simulink model "New_Controller"  (R2020b)
settings: Solver=VariableStepAuto  StartTime=0.0  StopTime=100  MaxStep=0.1  RelTol=1e-3
libraries: pid_lib x1
settings Model: Creator=Inver  LastModifiedBy=Inver

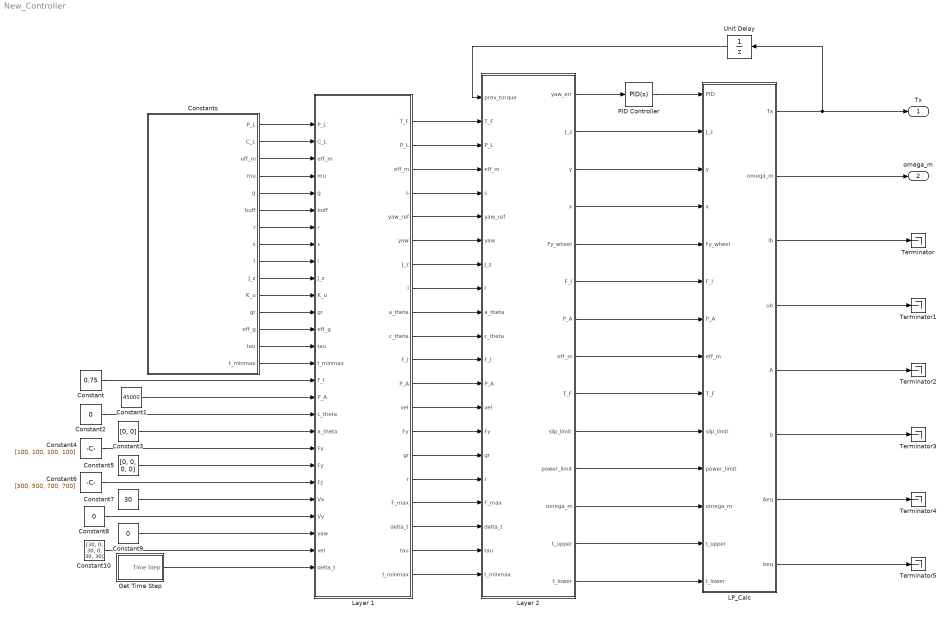
== system New_Controller ==
  Constant : Constant  Value=0.75
  Constant1 : Constant  Value=45000
  Constant10 : Constant  Value=[30, 0, 30, 0, 30, 30]
  Constant2 : Constant  Value=0
  Constant3 : Constant  Value=[0, 0]
  Constant4 : Constant  Value=[100, 100, 100, 100]
  Constant5 : Constant  Value=[0, 0, 0, 0]  VectorParams1D=off
  Constant6 : Constant  Value=[500, 500, 700, 700]
  Constant7 : Constant  Value=30
  Constant8 : Constant  Value=0
  Constant9 : Constant  Value=0
  "Constants " : MATLAB Function  TreatAsAtomicUnit=on
  Get Time Step : Subsystem
  "LP_Calc " : MATLAB Function  TreatAsAtomicUnit=on
  Layer 1 : MATLAB Function  TreatAsAtomicUnit=on
  Layer 2 : MATLAB Function  TreatAsAtomicUnit=on
  PID Controller : pid_lib/PID Controller  Controller=PID  Form=Parallel  TimeDomain=Continuous-time  UseExternalTs=off  SampleTime=-1  IntegratorMethod=Forward Euler  FilterMethod=Forward Euler  ControllerParametersSource=internal  P=40  I=3  D=0  UseFilter=on  N=100  TunerSelectOption=Transfer Function Based (PID Tuner App)  InitialConditionSource=internal  InitialConditionForIntegrator=0  InitialConditionForFilter=0  DifferentiatorICPrevScaledInput=0  ExternalReset=none  TrackingMode=off  Kt=1  LimitOutput=on  SatLimitsSource=internal  UpperSaturationLimit=inf  LowerSaturationLimit=-inf  LinearizeAsGain=on  AntiWindupMode=back-calculation  Kb=1  POutMin=[]  POutMax=[]  IOutMin=[]  IOutMax=[]  DOutMin=[]  DOutMax=[]  NOutMin=[]  NOutMax=[]  SumOutMin=[]  SumOutMax=[]  SaturationOutMin=[]  SaturationOutMax=[]  PParamMin=[]  PParamMax=[]  IParamMin=[]  IParamMax=[]  DParamMin=[]  DParamMax=[]  NParamMin=[]  NParamMax=[]  KbParamMin=[]  KbParamMax=[]  KtParamMin=[]  KtParamMax=[]  KbOutMin=[]  KbOutMax=[]  KtOutMin=[]  KtOutMax=[]  IntegratorOutMin=[]  IntegratorOutMax=[]  FilterOutMin=[]  FilterOutMax=[]  SumI1OutMin=[]  SumI1OutMax=[]  SumI2OutMin=[]  SumI2OutMax=[]  SumI3OutMin=[]  SumI3OutMax=[]  SumI4OutMin=[]  SumI4OutMax=[]  SumDOutMin=[]  SumDOutMax=[]  DifferentiatorOutMin=[]  DifferentiatorOutMax=[]  FilterDiffOutCoefMin=[]  FilterDiffOutCoefMax=[]  ReciprocalOutMin=[]  ReciprocalOutMax=[]  SumDenOutMin=[]  SumDenOutMax=[]  SumNumOutMin=[]  SumNumOutMax=[]  DivideOutMin=[]  DivideOutMax=[]  UdiffTsProdOutMin=[]  UdiffTsProdOutMax=[]  NTsProdOutMin=[]  NTsProdOutMax=[]  UintegralTsProdOutMin=[]  UintegralTsProdOutMax=[]  UngainTsProdOutMin=[]  UngainTsProdOutMax=[]  IntegratorContinuousStateAttributes=''  IntegratorStateMustResolveToSignalObject=off  IntegratorRTWStateStorageClass=Auto  FilterContinuousStateAttributes=''  FilterStateMustResolveToSignalObject=off  FilterRTWStateStorageClass=Auto  ParallelPVariant=InternalParameters  IdealPVariant=Disabled  IVariant=InternalParameters  DVariant=InternalParameters  IntegratorVariant=Continuous  SatVariant=Enabled  AWVariant=BackCalculation  PCopyVariant=Disabled  TRVariant=Disabled  FdbkBlocksVariant=Forward  IdealPFdbkVariant=Disabled  SatFdbkVariant=Disabled  DerivativeFilterVariant=ContFilter  NVariant=InternalParameters  NCopyVariant=Disabled  FilterICVariant=InternalICsFilter  IntegratorICVariant=InternalICs  ExternalResetVariant=Disabled  TRSumVariant=Passthrough  SumFdbkVariant=Disabled  SumVariant=Sum_PID  TsampFilterVariant=InternalTs  TsampNgainVariant=Passthrough  TsampIntegralVariant=Passthrough  ExternalSaturationOutDataTypeStr=Inherit: Same as second input
  Terminator{,1..5} (6 alike) : Terminator
  Unit Delay : UnitDelay  InitialCondition=[0; 0; 0; 0]  SampleTime=-1  HasFrameUpgradeWarning=on
  Tx : Outport
  omega_m : Outport  Port=2
  wires:
  Layer 1/15(gr) -> Layer 2/16(gr)
  Layer 1/14(Fy) -> Layer 2/15(Fy)
  "LP_Calc "/1(Tx) -> Unit Delay/1, Tx/1
  Layer 2/12(omega_m) -> "LP_Calc "/12("omega_m ")
  "Constants "/6(buff) -> Layer 1/6(buff)
  "Constants "/4(mu) -> Layer 1/4(mu)
  Layer 2/8(eff_m) -> "LP_Calc "/8(eff_m)
  Layer 2/13(t_upper) -> "LP_Calc "/13(t_upper)
  "LP_Calc "/7(Aeq) -> Terminator4/1
  "LP_Calc "/3(lb) -> Terminator/1
  "Constants "/3(eff_m) -> Layer 1/3("eff_m ")
  Layer 2/7(P_A) -> "LP_Calc "/7(P_A)
  "LP_Calc "/5(A) -> Terminator2/1
  Constant7/1 -> Layer 1/23(Vx)
  "LP_Calc "/6(b) -> Terminator3/1
  Layer 2/6(F_I) -> "LP_Calc "/6(F_I)
  Layer 2/10(slip_limit) -> "LP_Calc "/10(slip_limit)
  Layer 1/9(a_theta) -> Layer 2/10(a_theta)
  Layer 2/3(y) -> "LP_Calc "/3(y)
  "Constants "/13(eff_g) -> Layer 1/13(eff_g)
  "Constants "/11(K_u) -> Layer 1/11(K_u)
  Get Time Step/1(Time Step) -> Layer 1/27("delta_t ")
  "Constants "/14(tau) -> Layer 1/14("tau ")
  Constant2/1 -> Layer 1/18("c_theta ")
  Constant/1 -> Layer 1/16("F_I ")
  "LP_Calc "/2(omega_m) -> omega_m/1
  "Constants "/8(s) -> Layer 1/8("s ")
  Layer 1/3(eff_m) -> Layer 2/4("eff_m ")
  Layer 1/13(vel) -> Layer 2/14(vel)
  Constant4/1 -> Layer 1/20(Fx)
  Layer 1/20(t_minmax) -> Layer 2/21(t_minmax)
  Constant10/1 -> Layer 1/26("vel ")
  Layer 1/6(yaw) -> Layer 2/7(yaw)
  Layer 2/5(Fy_wheel) -> "LP_Calc "/5(Fy_wheel)
  Layer 1/4(s) -> Layer 2/5(s)
  Layer 2/9(T_F) -> "LP_Calc "/9(T_F)
  Layer 1/11(F_I) -> Layer 2/12("F_I ")
  "Constants "/12(gr) -> Layer 1/12("gr ")
  Constant3/1 -> Layer 1/19("a_theta ")
  "LP_Calc "/8(beq) -> Terminator5/1
  Layer 1/12(P_A) -> Layer 2/13("P_A ")
  "Constants "/1(P_L) -> Layer 1/1("P_L ")
  Unit Delay/1 -> Layer 2/1(prev_torque)
  Layer 1/7(J_z) -> Layer 2/8("J_z ")
  "Constants "/10(J_z) -> Layer 1/10("J_z ")
  Layer 2/2(J_z) -> "LP_Calc "/2(J_z)
  "Constants "/9(l) -> Layer 1/9("l ")
  Constant9/1 -> Layer 1/25("yaw ")
  Layer 1/5(yaw_ref) -> Layer 2/6(yaw_ref)
  "LP_Calc "/4(ub) -> Terminator1/1
  Constant1/1 -> Layer 1/17("P_A ")
  Layer 1/17(F_max) -> Layer 2/18(F_max)
  "Constants "/7(r) -> Layer 1/7("r ")
  Layer 1/16(r) -> Layer 2/17(r)
  Layer 2/14(t_lower) -> "LP_Calc "/14(t_lower)
  Layer 1/10(c_theta) -> Layer 2/11(c_theta)
  Constant5/1 -> Layer 1/21("Fy ")
  Layer 1/2(P_L) -> Layer 2/3(P_L)
  Constant6/1 -> Layer 1/22(Fz)
  "Constants "/5(g) -> Layer 1/5(g)
  Constant8/1 -> Layer 1/24(Vy)
  Layer 2/1(yaw_err) -> PID Controller/1
  "Constants "/2(C_L) -> Layer 1/2(C_L)
  Layer 1/18(delta_t) -> Layer 2/19(delta_t)
  "Constants "/15(t_minmax) -> Layer 1/15("t_minmax ")
  Layer 1/8(l) -> Layer 2/9(l)
  Layer 2/4(x) -> "LP_Calc "/4(x)
  Layer 1/19(tau) -> Layer 2/20(tau)
  Layer 2/11(power_limit) -> "LP_Calc "/11(power_limit)
  Layer 1/1(T_F) -> Layer 2/2("T_F ")
  PID Controller/1 -> "LP_Calc "/1(PID)

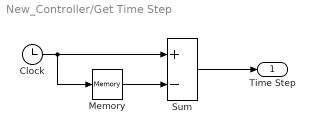
== system New_Controller/Get Time Step ==
  Clock : Clock
  Memory : Memory
  Sum : Sum  Inputs=+-
  Time Step : Outport
  wires:
  Memory/1 -> Sum/2
  Clock/1 -> Sum/1, Memory/1
  Sum/1 -> Time Step/1

== matlab function New_Controller/Layer 2 ==
  data: prev_torque input; yaw_err output; J_z output; T_F input; P_L input; eff_m input; s input; yaw_ref input; yaw input; J_z input; l input; a_theta input; c_theta input; F_I input; P_A input; vel input; Fy input; gr input; r input; F_max input; y output; x output; Fy_wheel output; F_I output; P_A output; eff_m output; T_F output; slip_limit output; power_limit output; omega_m output size=[1 4]; t_upper output; delta_t input; tau input; t_minmax input; t_lower output
function [yaw_err, J_z, y, x, Fy_wheel, F_I, P_A, eff_m, T_F, slip_limit, power_limit, omega_m, t_upper, t_lower] = Layer_2(prev_torque, T_F, P_L, eff_m, s, yaw_ref, yaw, J_z, l, a_theta, c_theta, F_I, P_A, vel, Fy, gr, r, F_max, delta_t, tau, t_minmax)
%% Calculations
% Calculate the Yaw Error, Apply Sign Convention
if yaw_ref(1) == 0 && yaw(1) == 0
    yaw_err = 0;
elseif c_theta >= 0
    yaw_err = min(abs(yaw_ref)) - yaw;
else
    yaw_err = (min(abs(yaw_ref)) * -1) - yaw;
end


% Motor Shaft Speed, RAD/S
omega_fl = sqrt((vel(1) * cos(a_theta(1)))^2 + (vel(2) * sin(a_theta(1)))^2);
omega_fr = sqrt((vel(3) * cos(a_theta(2)))^2 + (vel(4) * sin(a_theta(2)))^2);
omega_rl = vel(5);
omega_rr = vel(6);

omega_m = [omega_fl, omega_fr, omega_rl, omega_rr] .* (gr ./ r);


% Calculate K_1 Vehicle Constants
x_1 = (s(1) * cos(a_theta(1))) + (l(1) * sin(a_theta(1)));    
x_2 = (-1 * s(1) * cos(a_theta(2))) + (l(1) * sin(a_theta(2)));     
x_3 = s(2);     
x_4 = -s(2); 

x = [x_1, x_2, x_3, x_4]; 


% Transform Lateral Forces (Vehicle) to Lateral Forces (Wheel)
F_y_ij_fl = (sin(a_theta(1)) * Fy(1)) + (cos(a_theta(1)) * Fy(1));
F_y_ij_fr = (sin(a_theta(2)) * Fy(2)) + (cos(a_theta(2)) * Fy(2));
F_y_ij_rl = Fy(3);
F_y_ij_rr = Fy(4);

Fy_wheel = [F_y_ij_fl, F_y_ij_fr, F_y_ij_rl, F_y_ij_rr];


% Calculate K_2 Vehicle Constants
y_1 = (-1 * s(1) * sin(a_theta(1))) + (l(1) * cos(a_theta(1)));    
y_2 = (s(1) * sin(a_theta(2))) + (l(1) * cos(a_theta(2)));
y_3 = -l(2);
y_4 = -l(2);

y = [y_1, y_2, y_3, y_4]; 


% Torque Limits On Individual Wheels
Fx_max2 = (F_max.^2)-(Fy_wheel.^2);

% Control For Negative Output
for i = 1:4
    if Fx_max2(i) < 0
        Fx_max2(i) = 0;
    end
end

% Calculate Torque Limit Due to Power and Slip
Fx_max = sqrt(Fx_max2);
slip_limit = Fx_max ./ T_F; 
power_limit = (P_L .* eff_m) ./ omega_m;

% Control for large input
for i = 1:4
    if power_limit(i) > 15000
        power_limit(i) = 15000;
    end
end
 

% Calculate Constants for getting limit on motor output torque
e_term = exp(-delta_t / tau);
c_lower = (1 - e_term) .* t_minmax(1);
c_upper = (1 - e_term) .* t_minmax(2);
c_constant = (prev_torque .* e_term)';

% Max and Min Torque Limits
t_upper = max([c_upper + c_constant; c_constant + 1]);
t_lower = min([c_lower + c_constant; c_constant - 1]);


end

== matlab function New_Controller/LP_Calc  ==
  data: Tx output size=[4 1]; omega_m output; lb output double; PID input; J_z input; y input; x input; Fy_wheel input; F_I input; P_A input; eff_m input; T_F input; slip_limit input; power_limit input; omega_m input; t_upper input; ub output double; A output double; b output double; Aeq output double; beq output double; t_lower input
function [Tx, omega_m, lb, ub, A, b, Aeq, beq] = LP_calc(PID, J_z, y, x, Fy_wheel, F_I, P_A, eff_m, T_F, slip_limit, power_limit, omega_m, t_upper, t_lower)
%% Calculation
% Calculate Boundary Conditions
ub = [0, 0, 0, 0];
lb = [0, 0, 0, 0];

for i = 1:4
    ub(i) = min([slip_limit(i), power_limit(i), 25, t_upper(i)]);
    lb(i) = max(-1 * ub(i), t_lower(i));
end

% Calculate Yaw Constraint
Aeq = ((1 ./ J_z) .* x);
beq = PID-sum(((1 / J_z) * y) .* Fy_wheel);

% Calculate User Requested Torque Limit
A = [omega_m ./ eff_m; -1, -1, 1, 1];
b = [(F_I * P_A), sum(ub)];


%% Optimization
% Set Initial Guess
x0 = [5, 5, 5, 5];

% Set Optimization Parameters
options = optimoptions('fmincon','Algorithm','sqp');

% Maximize the Forces Acting on the Car
objfun = @(x) -(x(1) * T_F(1))-(x(2) * T_F(2))-(x(3) * T_F(3))-(x(4) * T_F(4));

% Find the Optimal Solution
Tx = fmincon(objfun,x0,A,b,Aeq,beq,lb,ub,[],options)';

end

== matlab function New_Controller/Constants  ==
  data: P_L output; C_L output; eff_m output; mu output; g output; buff output; r output; s output; l output; J_z output; K_u output; gr output; eff_g output; tau output; t_minmax output
function [P_L, C_L, eff_m, mu, g, buff, r, s, l, J_z, K_u, gr, eff_g, tau, t_minmax] = def_c()
%% Define Constants
% General Constants
mu = [1, 1, 1, 1]; % Maximum friction coefficient [Unitless]
g = 9.81; % Gravitational constant [m/s^2]
buff = 0.05; % Buffer value when calculating max allowable yaw

% Motor Constants
P_L = [15, 15, 15, 15] * 1000; % Power limit for each motor [W] 
C_L = [70, 70, 70, 70]; % Current limit for each motor [Amp]
eff_m = 0.85; % Motor efficiency [Unitless]
tau = 0.02; % Motor Response Time Constant
t_minmax = [-25, 25]; % Minimum and maximum torque you can request from motor

% General Vehicle Constants
r = 0.3; % Tire radius [m]
s = [1, 1]; % Half track width [m]
l = [1, 1]; % Wheelbase [m]
J_z = 4000; % Polar moment of inertia [kg m^2]
K_u = 0.05; % Understeer gradient

% Gearbox Constants
GR_f = (37/24) * (84/23) + 1; % Front gear ratio [Unitless]
GR_r = (40/21) * (84/23) + 1; % Rear gear ratio [Unitless]
gr = [GR_f, GR_f, GR_r, GR_r]; % Gear ratios [Unitless]
eff_g = 0.97; % Gearbox power transmission efficiency [Unitless]


end

== matlab function New_Controller/Layer 1 ==
  data: T_F output; P_L output; eff_m output; s output; yaw_ref output; yaw output; J_z output; l output; a_theta output; c_theta output; F_I output; P_A output; vel output; Fy output; gr output; r output; F_max output; P_L input; C_L input; eff_m input; mu input; g input; buff input; r input; s input; l input; J_z input; K_u input; gr input; eff_g input; tau input; t_minmax input; F_I input; P_A input; c_theta input; a_theta input; Fx input; Fy input; Fz input; Vx input; Vy input; yaw input; vel input; delta_t input; delta_t output; tau output; t_minmax output
function [T_F, P_L, eff_m, s, yaw_ref, yaw, J_z, l, a_theta, c_theta, F_I, P_A, vel, Fy, gr, r, F_max, delta_t, tau, t_minmax] = Layer_1(P_L, C_L, eff_m, mu, g, buff, r, s, l, J_z, K_u, gr, eff_g, tau, t_minmax, F_I, P_A, c_theta, a_theta, Fx, Fy, Fz, Vx, Vy, yaw, vel, delta_t)
%% Calculation
% Max Allowed Force On Each Wheel
F_max = abs(mu'.*Fz)';

% Convert Torque At The Motor Shaft to Force At The Wheel
T_F = (gr .* eff_g) ./ r;


% Yaw Calculations
v_cog = sqrt(Vx^2 + Vy^2);
yaw_des = (v_cog * abs(c_theta)) / ((l(1) + l(2)) + (K_u * v_cog ^ 2));
yaw_max = (max(mu) * g) / (v_cog + buff);
yaw_ref = [yaw_des, yaw_max];

end
